simulink model "PART_1_2_FIRSTPRINCIPLESANDBLACKBOXMODEL"  (R2024a)
settings: Solver=VariableStepAuto  StartTime=0.0  StopTime=10  RelTol=1e-3
libraries: arduino_io_lib x4
settings Model: Creator=Çağlar  LastModifiedBy=Çağlar

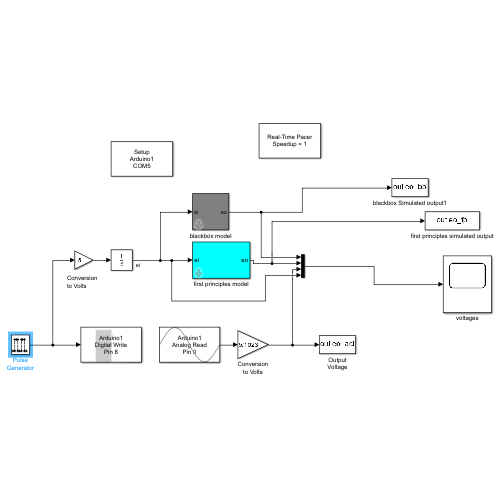
[thumbnail: Simulink's stored preview of the top-level diagram]
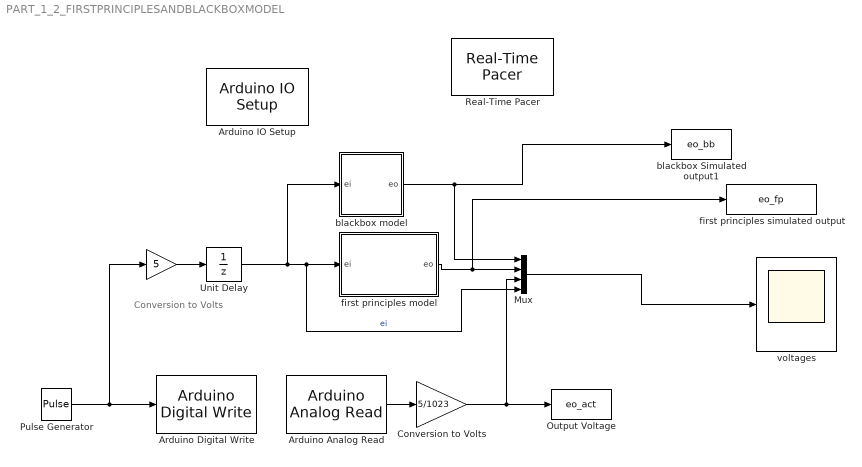
== system PART_1_2_FIRSTPRINCIPLESANDBLACKBOXMODEL ==
  note: Conversion
      | to Volts
  " " : Gain  Gain=5
  Arduino Analog Read : arduino_io_lib/Arduino Analog Read  arduinoVar=Temporary arduino variable: Arduino1  arduinoPin=0  T=0.05
      settings: SourceProductName=Arduino IO Library
  Arduino Digital Write : arduino_io_lib/Arduino Digital Write  arduinoVar=Temporary arduino variable: Arduino1  arduinoPin=8  T=-1
      settings: SourceProductName=Arduino IO Library
  Arduino IO Setup : arduino_io_lib/Arduino IO Setup  Priority=3  arduinoVar=Temporary arduino variable: Arduino1  workspaceVarName=b  comPort=COM5
      settings: SourceProductName=Arduino IO Library
  Conversion to Volts : Gain  Gain=5/1023
  Mux : Mux
  Output Voltage : ToWorkspace  VariableName=eo_act  SampleTime=-1
  Pulse Generator : DiscretePulseGenerator  Period=2000  PulseWidth=100  PhaseDelay=1  SampleTime=0.05
  Real-Time Pacer : arduino_io_lib/Real-Time Pacer  simTimePerRealTime=1
      settings: SourceProductName=Arduino IO Library
  Unit Delay : UnitDelay  SampleTime=-1  HasFrameUpgradeWarning=on
  blackbox Simulated output1 : ToWorkspace  VariableName=eo_bb  SampleTime=-1
  blackbox model : Subsystem  mask{K=1, tau=0.79}
  first principles model : Subsystem  mask{R=15*10^3, C=56*(10^-6), q_init=0}
      mask prompts: R "Resistance"; C "Capacitance"; q_init "Initial charge on capacitor"
      mask Display:
      | port_label('input', 1, 'ei');
      | port_label('output', 1, 'eo');
  first principles simulated output : ToWorkspace  VariableName=eo_fp  SampleTime=-1
  voltages : Scope
  wires:
  Pulse Generator/1 -> " "/1, Arduino Digital Write/1
  Arduino Analog Read/1 -> Conversion to Volts/1
  Mux/1 -> voltages/1
  " "/1 -> Unit Delay/1
  first principles model/1(eo) -> first principles simulated output/1, Mux/2
  Unit Delay/1 -> blackbox model/1(ei), Mux/4, first principles model/1(ei)  "ei"
  blackbox model/1(eo) -> Mux/1, blackbox Simulated output1/1
  Conversion to Volts/1 -> Mux/3, Output Voltage/1

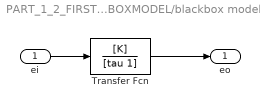
== system PART_1_2_FIRSTPRINCIPLESANDBLACKBOXMODEL/blackbox model ==
  ei : Inport
  Transfer Fcn : TransferFcn  Numerator=[K]  Denominator=[tau 1]
  eo : Outport
  wires:
  ei/1 -> Transfer Fcn/1
  Transfer Fcn/1 -> eo/1

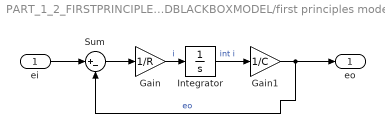
== system PART_1_2_FIRSTPRINCIPLESANDBLACKBOXMODEL/first principles model ==
  ei : Inport
  Gain : Gain  Gain=1/R
  Gain1 : Gain  Gain=1/C
  Integrator : Integrator  InitialCondition=q_init
  Sum : Sum  Inputs=|+-
  eo : Outport
  wires:
  Gain1/1 -> eo/1, Sum/2  "eo"
  ei/1 -> Sum/1
  Sum/1 -> Gain/1
  Integrator/1 -> Gain1/1  "int i"
  Gain/1 -> Integrator/1  "i"
